simulink model "MicrowaveNoActions"  (Simulink 9.0)
settings: Solver=ode45  StartTime=0.0  StopTime=20  RelTol=1e-3  EnableMultiTasking=on
settings Model: SuppressorTable=22 serialization::archive 11 0 6 0 0 0 0 0  Creator=bourbouh  LastModifiedBy=hbourbou
settings DataIOCC: LimitDataPoints=on  SaveFormat=Structure
settings DebuggingCC: UnderspecifiedInitializationDetection=Simplified  MergeDetectMultiDrivingBlocksExec=error
settings GRTTargetCC: GeneratePreprocessorConditionals=Disable all

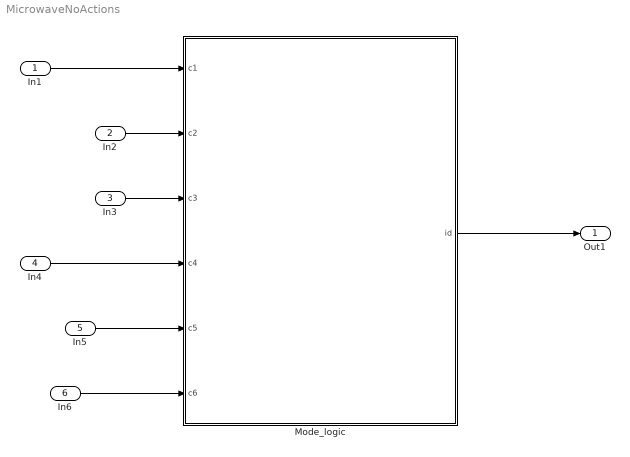
== system MicrowaveNoActions ==
  In1 : Inport  OutDataTypeStr=boolean
  In2 : Inport  Port=2  OutDataTypeStr=boolean
  In3 : Inport  Port=3  OutDataTypeStr=boolean
  In4 : Inport  Port=4  OutDataTypeStr=boolean
  In5 : Inport  Port=5  OutDataTypeStr=boolean
  In6 : Inport  Port=6  OutDataTypeStr=boolean
  Mode_logic : Stateflow chart  TreatAsAtomicUnit=on
  Out1 : Outport
  wires:
  Mode_logic/1(id) -> Out1/1
  In1/1 -> Mode_logic/1(c1)
  In6/1 -> Mode_logic/6(c6)
  In5/1 -> Mode_logic/5(c5)
  In4/1 -> Mode_logic/4(c4)
  In3/1 -> Mode_logic/3(c3)
  In2/1 -> Mode_logic/2(c2)

== stateflow chart Mode_logic ==
  settings: updateMethod=DISCRETE  sampleTime=1
  state SETUP
    en: id=1;
  state RUNNING
    state COOKING
      entry: id=2;
    state SUSPENDED
      entry: id=3;
    COOKING -> COOKING [order 1] : [c4]
    (default) -> (junction 7)
    (junction 7) -> COOKING [order 1] : [c5]
    (junction 7) -> SUSPENDED [order 2]
    SUSPENDED -> COOKING [order 2] : [c6]
    COOKING -> SUSPENDED [order 2] : [c6]
  (default) -> SETUP
  SETUP -> (junction 21) : [c1]
  (junction 21) -> RUNNING : [c2]
  (junction 22) -> SETUP
  RUNNING -> (junction 22) : [c3]
  SUSPENDED -> (junction 22) [order 1] : [c4]
  data: c1 input boolean; c2 input boolean; c3 input boolean; c4 input boolean; c5 input boolean; c6 input boolean; id output double
